simulink model "reactor_simulink"  (R2018a)
settings: Solver=ode15s  StartTime=0.0  StopTime=10  FixedStep=0.01  MaxStep=5  RelTol=1e-6  EnableMultiTasking=on
settings Model: Creator=mb27748  LastModifiedBy=kr27867
settings DataIOCC: SaveFormat=Array  SignalLogging=off  DSMLogging=off  VisualizeSimOutput=off  SaveTime=off  TimeSaveName=tout_nl
settings OptimizationCC: LifeSpan=inf
settings DebuggingCC: UnderspecifiedInitializationDetection=Classic  MergeDetectMultiDrivingBlocksExec=none  SolverPrmCheckMsg=warning  SFUnexpectedBacktrackingDiag=warning  SFNoUnconditionalDefaultTransitionDiag=warning  SFExecutionAtInitializationDiag=none
settings HardwareCC: ProdBitPerPointer=32  ProdBitPerSizeT=32  ProdBitPerPtrDiffT=32  ProdLargestAtomicFloat=None  ProdIntDivRoundTo=Undefined  ProdEndianess=Unspecified  ProdWordSize=32  ProdHWDeviceType=32-bit Generic
settings ModelReferenceCC: PropagateSignalLabelsOutOfModel=off
settings CodeAppCC: StateflowObjectComments=on
settings GRTTargetCC: TargetLangStandard=C89/C90 (ANSI)  GeneratePreprocessorConditionals=Disable all
settings ConfigComp: CovMetricSettings=dw  CovHtmlReporting=on  CovSaveCumulativeToWorkspaceVar=on  CovSaveSingleToWorkspaceVar=on  CovExternalEMLEnable=off  CovSFcnEnable=off

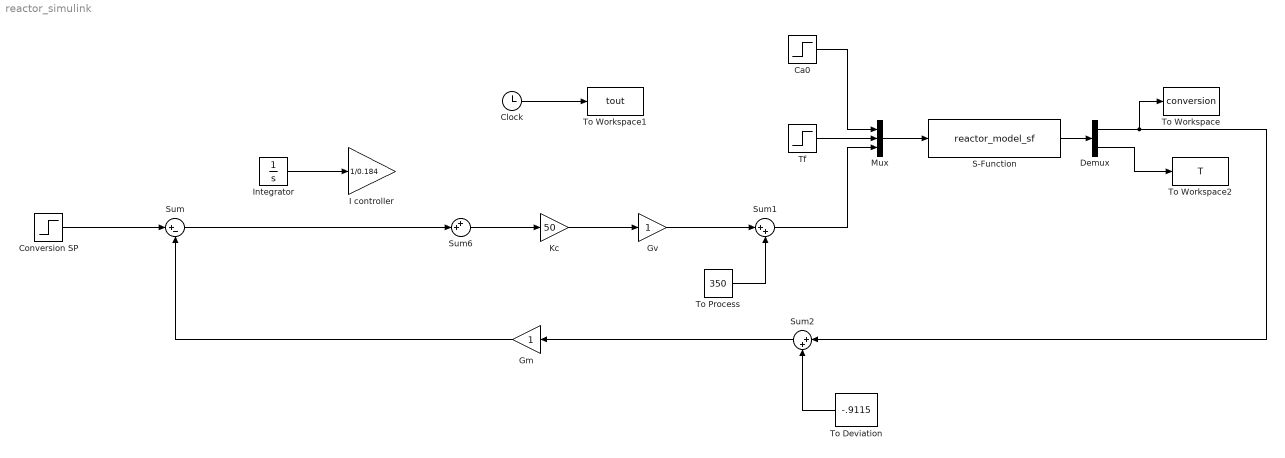
== system reactor_simulink ==
  "Ca0 " : Step  Time=0  Before=1  After=.99  SampleTime=0
  Clock : Clock
  Conversion SP : Step  Time=0  After=0  SampleTime=0
  Demux : Demux  Outputs=2
  Gm : Gain
  Gv : Gain
  I controller : Gain  Gain=1/0.184
  Integrator : Integrator
  Kc : Gain  Gain=50
  Mux : Mux  Inputs=3
  S-Function : S-Function  FunctionName=reactor_model_sf  SFunctionDeploymentMode=off  EnableBusSupport=off
  Sum : Sum  Inputs=|+-
  Sum1 : Sum  Inputs=|++
  Sum2 : Sum  Inputs=|++
  Sum6 : Sum  Inputs=++|
  "Tf " : Step  Time=0  Before=350  After=345  SampleTime=0
  To Deviation : Constant  Value=-.9115
  To Process : Constant  Value=350
  To Workspace : ToWorkspace  VariableName=conversion  SampleTime=-1
  To Workspace1 : ToWorkspace  VariableName=tout  SampleTime=-1
  To Workspace2 : ToWorkspace  VariableName=T  SampleTime=-1
  wires:
  Clock/1 -> To Workspace1/1
  "Ca0 "/1 -> Mux/1
  "Tf "/1 -> Mux/2
  Mux/1 -> S-Function/1
  S-Function/1 -> Demux/1
  Demux/1 -> Sum2/1, To Workspace/1
  Demux/2 -> To Workspace2/1
  Kc/1 -> Gv/1
  Sum2/1 -> Gm/1
  Sum1/1 -> Mux/3
  To Process/1 -> Sum1/2
  To Deviation/1 -> Sum2/2
  Integrator/1 -> I controller/1
  Sum6/1 -> Kc/1
  Gv/1 -> Sum1/1
  Conversion SP/1 -> Sum/1
  Gm/1 -> Sum/2
  Sum/1 -> Sum6/2
